simulink model "LCL_filter_blok_schem_S"  (R2021b)
settings: Solver=VariableStepAuto  StartTime=0.0  StopTime=Tsim  RelTol=1e-3
model workspace (MAT data in the model file):
  C = sym
  C.s = 'symobj::fromString("eJytU0tOwzAQddqUryqBBEJ0FQlOwAnKZ8MSumMTOWQogxxHZJyi7DgFd4JTYU8r6rhpxaKWXjKacd6bebH7QoieEJ9f9h33o4F9jUdivvo2PlnEdo/Yd6CGJBFONadb9SuHD8AqT2ayQpkpSLQsgJKaIE9QJ9QUZfZ2VxdFc5+DNviCUAlfsxdwxg6vpcpt/szbM+qIw375W1KlCfI7DmRyhRlrH4jlGjoQmElTXCuUBDSf89zT+BGttVZ/1yH9c6tVO3VYa8eSc9A5U53ZtsbfXhOHG/rgeVN4r6Vi7kvPu4tFHHV46fPHAeeeA5VqBuxiy0Ou3UjC5wmYgOco2MvzVOA6a/EzHtMVf32uYTCLXzsOdPhfoDYwZYdXtZ62p8XzV9Jgqbvneki3d+n+e5A2XSw/7w5CdGsfvwMla0g=", 2)'
  C.Digits = 32
  Cx = 3
  F = tf
  F.IOSize_ = [1 1]
  F.Data_ = ltipack.tfdata
  F.Data_.num = {[0 6e-06 0 0 0]}
  F.Data_.den = {[-3e-09 -9e-06 0.06 0.0002 1]}
  F.Data_.Delay.Input = 0
  F.Data_.Delay.Output = 0
  F.Data_.Delay.IO = 0
  F.Data_.Ts = 0
  I2 = sym
  I2.s = 'symobj::fromString("eJytVEtOwzAQdZqEfmgpf0RXkeAC9ATls0FiQys2bKKUmGLkJCVOWmXHKbgTXApiN1Bn4kRUraWRPePJm3nPdnSEUA2h9490NnTNTKdBDy2Gnq4Ps3Wag5rcWMIcxsjEF+Hcfp/bHJPQtWZOSJwxxZbveJhZMcOuRXyLJV4wfr2JPS+5dbEfkWeCQyTXrAFMg9tLQN00fiLl9BRr2K/4ltEgAvEtbixyKRmL2i20HB1uDEejxLukxGGYLXieSjW+UG6U1q9zs//Uyu0dcSuVY4lpKjnF47StwafUxHZFH4Kvjd9ihwrsc0m7s2ytKbSU8Q2A2eDGAjrDQsWchmLvymHkaYQjgLMLcgWfEPPOcvjChnZBXxmrA7jIe3ugjjgL4kd4IhQu1nrcXC3BP3QiEvhqXvf25h7dfy9S1cP6zamDHN6YaXsxjYp1+YXRrotxYXcXJfG+Guch36v6Ak+DefazKHyfPVIdLYeWOVrFoTalvYaS+5TGrNhb1cNYXNwS/sN+DstQYMn+FvC7wG9JWDAXYpkK7CpdZL8Ota1l8woYLYhhLDFycX6g3+lYg9sB8HeA3wb+8Zo6Qq2qzqy9wVqQV3fF85D9/TX6gpxVfcl+D+r/AxkWrVk=", 2)'
  I2.Digits = 32
  L1 = sym
  L1.s = 'symobj::fromString("eJytU8tOwzAQ3DYpT1UCCYToKRL8AHxBQVyQuJTeuEQOWYqRk4isU5QbX8E/wVdhbyvqOGnFoZZGWXmdmZ1JHABAH+DzyzzDoDcwj/EIFisw9cmyNmdg34JqEkRylvN2o39t8YGyTKO5KKVIFEa5yJCiijCNZB5RnRXJ212VZfV9irmWLxJLcDX7Hmdo8Vqo1OyfOWdGHbU/L79LqtDe/o4F6VTJhLUPYLWGFoR6Wmc3SgpCWvg8dzR+oLHW6u9axH9pNXqnFmvjWHEOOj1ViRlr/O0McbhhDvYb43slFHNfOtldLOteR5Yuf+hx7llQoebIKTYy5N6tIPk8Re3xHHln2U+JdrIGP+MxbuXrcg09L27v2NPhbyFzjTNOuK31tD0t9l8KLYu829ck3t6l+++PtOlitQZ8uAL4BQPqa4Q=", 2)'
  L1.Digits = 32
  L1x = 0.01
  L2 = sym
  L2.s = 'symobj::fromString("eJytU8tOwzAQdNuUpyqBBEL0FAm+gC8oiAsSF+iNS+SQpSxyHJF1inLjK/gn+CrsbUUdJ6041NIoK68zszOJB0KIvhCfX/YZDXpD+5iMxWINbH2yrO0Zse9ANUkinGnebvSvHD4AyyyeyxJlqiDWMgeKK4IsRh1TnRfp222V5/VdBtrgC0IpfM1+wBk5vBYqs/tn3plxRx3Oy++SKkywv+NAJlOYsvaBWK2RA4GZ1vm1QklAC5/nnsaPaKy1+rsOyV9ajd6pw9o4VpzDTk9VaseafHtDHG6Yg/0m8F5JxdyXXnYXy7rXkaXPHwWcew5UqDlwio0MuXcjCZ+nYAKeo+As+ynBTdbgZzwmrXx9rlHgxe8dBzr8LVAbmHHCba2n7Wmx/1IaLHS3r4dke5fuvz/SpovVGvDeXuVfA+1rhQ==", 2)'
  L2.Digits = 32
  L2x = 0.01
  R1 = sym
  R1.s = 'symobj::fromString("eJytU8tOwzAQ3LYpT1UCCYToKRL8AHxBQVw4Qm9cIocsxchxRNYpyo2v4J/gq7C3FXWctOJQS6OsvM7MziQeAEAf4PPLPqNBb2gfkzEs1sDWJ8vanoF9B6pJEMmZ5u1G/9rhA2WZxXNRSpEqjLXIkeKKMIuljqnOi/Ttrsrz+j5DbeSLxBJ8zX7AGTm8Fiqz+2femXFHHc7L75IqTLC/40AmUzJl7QNYrZEDoZnW+Y2SgpAWPs89jR9orLX6uw7JX1qN3qnD2jhWnMNOT1Vqx5p8e0McbpiD/Sb4XgnF3JdedhfLuteRpc8fBZx7DlSoOXKKjQy5dytIPk/RBDxHwVn2U6KbrMHPeExa+fpco8CL3zsOdPhbSG1wxgm3tZ62p8X+S2Fkobt9PSTbu3T//ZE2Xax28FcAvwQCa4o=", 2)'
  R1.Digits = 32
  R1x = 50
  R2 = sym
  R2.s = 'symobj::fromString("eJytU8tOwzAQdNuUpyqBBEL0FAm+gC8oiAtH6K2XyCFLWeQ4IusU5cZX8E/wVdjbijpOWnGopVFWXmdmZxIPhBB9IT6/7DMa9Ib2MRmL5RrY+mxV2zPi0IFqkkQ417zd6N84fACWWbyQJcpUQaxlDhRXBFmMOqY6L9K3+yrP64cMtMEXhFL4mv2AM3J4LVRm9y+8M+OOOpyX3yVVmGB/z4FMpjBl7SOxXiMHAjOt81uFkoCWPi89jR/RWBv19x2Sv7QavXOHjXGsOYednqrUjjX59oY43jIH+03gvZKKua+97K5Wda8jS58/CjgPHKhQC+AUGxly704SPk/BBDwnwVn2U4KbrMHPeEpa+fpco8CL3zsNdPhboDYw54TbWrPdabH/UhosdLevx2R3l+6/P9K2i9UO3l7lXwQFa4s=", 2)'
  R2.Digits = 32
  R2x = 20
  Tchirp = 0.04
  Tsim = 0.05
  Tstep = 0.02
  U = sym
  U.s = 'symobj::fromString("eJytU0tOwzAQddqUryqBBEJ0FQlOwAkKYsMSKjZsIocMZZDjiIxTlB2n4E5wKuxpRR03rVjU0ktGM857My92XwjRE+Lzy77jfjSwr/FIzFffxieL2O4R+w7UkCTCqeZ0q37l8AFY5clMVigzBYmWBVBSE+QJ6oSaoszebuuiaO5y0AZfECrha/YCztjhtVS5zZ95e0Ydcdgvf0uqNEF+x4FMrjBj7QOxXEMHAjNpimuFkoDmc557Gj+itdbq7zqkf261aqcOa+1Ycg46Z6oz29b422vicEMfPG8K77VUzH3peXexiKMOL33+OODcc6BSzYBdbHnItRtJ+DwBE/AcBXt5ngpcZy1+xkO64q/PNQxm8WvHgQ7/C9QGpuzwqtbT9rR4/koaLHX3XPfp9i7dfw/Spovl591BiB7t4xcDbWta", 2)'
  U.Digits = 32
  UR2 = sym
  UR2.s = 'symobj::fromString("eJytVEtOwzAQddq0Da0q/iC6igQXoCconw0SG1qxYROlxBQjJymx0yo7TsGd4FIQu4E6EydQtZZG8YzHb+Y926kjhGoIvb2nX7NuNNLPoIcWo57OD7J5moO2hLGEuYyRSSDDufW+sDkmkWfP3Ii4Y4rtwPUxs2OGPZsENkv8cPxyHft+cuPhgJMngiOk1qwBTFPYc0i9NH6s5PQ0c9iv3MtoyEG8KYxxj5KxrN1Gy9EVxjAfJf4FJS7DbMHzRKnxiXKjtH5LmPOrVm7tUFipHEvMhpZTPE7bGnwoTXQq+pB8Hfwau1RinynanWZzQ6Olim8CTEsYC+kMSxVzGsq1S5eRxxHmAGcH5Eo+ERad5fClDZ2CvipWF3BR13ZBHXkWJOB4IhUu1nrYXC3JP3I5CQM9rztnc4/uvxep6mH95FggRzTWcPyY8mJdcWGMq2Jc2u15Sbyvjw+LcYl/n+egv9jTcJ79RAr7s8dbR8thZI5RcdjtPzWZ0pgVe6t6MAueC13UPEvBMDUYqt/U7C37CcBciNXQYFfpofotqGkt+66A0YEY5hIjFxcH+ZWONbjtA39b87hV/2hNHaFWVWfW3WAtyMta8TxUf2+NviBnXV+q34P6fwPdPq5b", 2)'
  UR2.Digits = 32
  Ux = 10
  Z = sym
  Z.s = 'symobj::fromString("eJzNWN1O1EAUntJdERXERIMgxlW440a5xJgsgiQkEiPcGBSbWTq7jOkfnRYoV1z6BL6TPpMJdqaFnZ6ZTncNFzSZtGdm+p2/75zOro0QmkDo4ld+b9lWO791F1Bx2fnz4/I534Om+GAZw4zRQSCmK+urfJwSGrudExxT3PNIJ8A+YZ2UEbdDgw7L/LD3YzP1/WzbJUFC+5TESNY5ATBbfByFnpvPz0l7FjTP0F7xLvPCBMzf4YMlrkd7Qvc9NLym+WAk2cv8dY9iRljh57yk4w+qXLX6J/lwrqNVWXvCR204hphtrU9pLzer+1sy4r7BDuGvQ45T7AnsZSl2S+WzpYmljN8CmHf5YKF3QkQUKzEUa+8xo4d7JAE4s2Cv8Ccm3LIKvhi7jhJfGWsa+CKvPQJ6RC5okJCBiLCqa//mdAn/Y5zQMND79dm5uaIblUimwrpyrGUgxP8Ums3HZugjECBByB2cxPRM2GgioYmQstwGOh7y8eEsikkeuDDYooS7irrPhnhC94shHtffyte7M0OYCqZIHnXFPCw+iLOTz9lIuZT3ZPmBodHYOkJvhDmjg4Tjvizn8wJDPwsbkGvImSCpQ/IAMXKsy9unVOAqeXZxgg3NBzYKgeXQPjLsKWzx8HnmhPEYjUyOr2WVd938ZX4ZuDTXVCdBGPGGu3iFWYPztKmOCx9xICjUlBuPlJ4qOmT5ucGvjmavqfnL/OI8mi0+kmtr20GfBjTJxvhAmD6ywj8J0xRDkz6YD+iDsGEDR5GXCRtG7SUrWhzqFqVWzxUxwkjRpdSDj/mm6wONBTBlW14DeVFja12PHsdH0U/yfG2lwSFq0AkPGyYe1PXM2YZeeBtk5aDi0n5f7rWXlxdyr5X95nNWHyl+mw5qso66+EI+rBjqR9vLcDxgjT02xsGACNsrvXSivBv4ug7kmTG5I8tvgfzuFnBibM4kWUTAPv6dbziHWH8bsEWeKDsncSjeH+U80pQXWeb7684iFti7rXm3LsdTmhwr/JP8quPZpLQG7ZmCvLX1+/alHsztfDV8vq7hK5xSrj3D8EN82/FTT3wiND3w4xtlXvSI8gembNe8oT4LPZGXsho9u4Weuvh/BfI3IB/oesaS88UB8bFBfKSYVWIEdatxWVX8PzDEA2I6QMZj+A7r8qDhXXPPjMLT8s8MJccbSPER5lheOxohHrL8HciHDVwu5zTcUXPRh9j/AGWyXjA=", 2)'
  Z.Digits = 32
  ZI3 = sym
  ZI3.s = 'symobj::fromString("eJzNWN1O1EAUntJFRAUx0SCIcRXvuFEuMSaLIAmJxAgxMSg2s9vZZUz/6LRAueLSJ/Cd9JlMsDMt7PTMdLpruGCSk86ZmX7n/3R2bYTQBELnv/Jny7Ym80dnERXDzucPy3l+Bk1zYhnDjNFBIJYr+6ucTgiN3fYxjinueqQdYJ+wdsqI26ZBm2V+2P2xmfp+tu2SIKF9SmIky5wAmC1Oh6Hn5uvz0plFzRzqK95lXpiA9VucWOJ6tCtk30HDMcOJkWQv89c9ihlhhZ0Lkow/qDJq5U9xcq68Vdl7xKnWHUPMSa1NaTdXq/NbUuKuQQ9hr0OOUuwJ7JeS75bLuaXxpYzfApi3ObHQOybCixUfir13mNHeHkkAzhw4K+yJCdesgi9o11H8K2PNAFvkvQdAjogFDRIyEB5WZe1fnyxhf4wTGgZ6uz4511d0oyaSqbAuDWsZEuJ/Cs3mtBn6CDhIJOQOTmJ6KnQ0JaEpIWV+Esi4z+n9aRST3HFhsEUJNxV1ngzxhOxnQzwuv5Xvd2aHMBVMETzqinVYfBBnJ1+zkTKU92T+nqHR2LqE3gjzjA4Sjvu8XM8LDP0sdECuIWYiSR2SO4iRI13cPqYCV4mzixNsaD6wUQgsh/aR4Uyhi4fPMieMx2hksn8tq3zq1i/yYcil+aY6CcKIN9ylS8wanMdNdVzYiAORQk2x8UhpqSJD5p8a7Gprzpqav5xfPI/mio/k2tp20KcBTbIxPhCmj6ywT8I0+dAkD8YD2iB02MBR5GVCh1F7yYoWh7pFqdXniqAwUmQp9eBjfujqQmMBTFmXV4Bf0uha16PHsVH0kzxeW2nQQw0y4WXDlAd1PXOuoRfeBF65qLi035d77cXFudxrZbv5mtVHit2mi5oso86/MB9WDPWj7WU4HrDGHhvjYECE7pVeOlE+Dfm6DvjZMXNH5t8A/u0NyImxcybJIgLO8e98wz3E+tuALeJE2RmJQ/H+KPeRprjIPD9fdxexwNltzbt1MZ7WxFjJP8muujybkvagPtMwb239uX2pB3M9XwznVzV8iVPytXcYfomfdPzUE58ITQ/88FpZFz2i/IEp67VgqM9CTuSlrEbObiGnzv9fAf8N8Ae6nrHsfHGAf2zgH8lnFR9B2apfVhX7Dwz+gJgO4PEYtsO6PGh419wzo/Ck/DNDifEGUmyEMZb3Dkfwh8x/B3wPxMpC1VhZOh0/qzr2/gEclVyL", 2)'
  ZI3.Digits = 32
  a = [-3e-06 -0.009 60 0.2 1000]
  b = [0.006 0 0 0]
  cit = sym
  cit.s = 'symobj::fromString("eJytU0tOwzAQdZqEryqBBEJ0FQlOwAkCYsMSuusmcshQjJwEMk6r7DgFd4LzcABsJ1DbTSoWtfTk8YzzZubF4xNCRoS8f8g98L1QbvGEtMuX9klnyztkXwEbpIhsXmi3Fb9SWAKrsmhBK0ZTDlFBc8CoRsgiVkTY5GX6clvneXOXQSHYE4OKmDlHDmeg8FzyTPrPjDuTHtutV3+LvBSOf0cBRcZZqnMfkNUaKyCIaZNfc0YRsO3z3MjxRaw1mH9XIflTy4qdKgzKseIMe3uqU1lW/GkUcbihDt1vAm815Zr70tDuorO9Hi1N/sDh3FPAki9Aq2hpqGM3FNnjFITDc+Tc1f1UoCqz+DUekjV9Ta6x04sZO3by6H/BCgFzrfB6rtn2cun+KypYWfT3dZ9sb+j++5A2DdZQblVYmOQ1FzZX/wN7LZfdMJsx9bC8boh8QySvO8h4HJj+39i3155/AKW1cyg=", 2)'
  cit.Digits = 32
  color = 'r'
  men = sym
  men.s = 'symobj::fromString("eJy1VN1OgzAULgOm0yxqojHuikSfwGsv5uKNl7o7b0iROmsKTE7Zwp1P4Tvpk+wttC1MSmGbJrPJCeX8fN85Hy02QqiD0Nu7eDq25YrHcICKZYv9cbkXOagnDXLAAHQSK3ctfiltTmgaejOcUhww4sU4IuBlQEKPxh7kURK83GRRlN+GJOb0iZIU6ZwdA9OR9pywUPhPtZxBy97sV9UCS7jh70oDHjIaKO49VK2+NCB8nEfXjGIgUMx5pnF8otpayb8jzf9RqxY7kbZSjgrTbZ0pC0Rbww+tif01fah5ffKaYaawLzTtzsu91aKlju8YmLvSIGEzolSsaahiIwz0cUy4gXNo5Kp5UiI7q+Eru/cb+upYfWMWPXZk8KhvQWNOJkrhJtfD9rjU/CnmNInb57rzt3fpfnuQ1l2sZU7XyJGNuf6UZVDHMnss8qKM8WZ/8mBZZb2jiaT8VllcvK8U3914uKfJvPyR6HVyHlvn7FRcNf/V33vQY71NvHaF39BAfuCFSPgS67/4nTX8MnE4Oljy1+oWxZv1DVG6i7I=", 2)'
  men.Digits = 32
  s = sym
  s.s = 'symobj::fromString("eJytU0tOwzAQddqUryqBBEJ0FQlOwAkKYsMSuusmcshQBjmOyDhF2XEK7gSnwp5W1HHTikUtPXk047yZ92L3hRA9IT6/7B73o4HdxiOxWH0bny1je0YcOlBDkghnmtOt+o3DB2CVJ3NZocwUJFoWQElNkCeoE2qKMnu7r4uiechBG3xBqITfsxdwxg6vpcpt/sI7M+qIw3n5W1KlCfJ7DmRyhRn3PhKrNXQgMJOmuFUoCWih89Lr8SNaa2P/fYf0z61W7dxhox0rzkGnpjqzY42/vSGOt8zBelN4r6Vi7mvPu6tlHHV46fPHAeeBA5VqDuxiy0Ou3UnC5wmYgOckOMt6KnCTtfgZT+mavz7XMNDi106DPvwvUBuYscPrvaa768X6K2mw1N26HtPdPbr/XqRtD8vPu4sQuUv/CwPla3g=", 2)'
  s.Digits = 32
  sim = 'HPF'
  u = sym
  u.s = 'symobj::fromString("eJzNVk9P1EAUn9JFXBXERAMixlW8cTEeMSaLIAkHYpSYGC/NLJ1dx7TTpdNFyomjn8DvpJ/JZJ15Xdjp63TKGg5M8tLOn/7ev997HZ8QMkfI+S/1bPnevHp010gxfPX+cPKuzpC2FplLKiUfCFgu7b/W8oPxNOyc0JTTXsQ6gsZMdkaShR0uOjKPk9733VEc5/shExnvc5YSU+ccwmxp+ZZEoVpfMc6sWd6xvfCtjJIMrd/SIrMw4j3QfYdMx6IWybLDPN6OOJVMFn4+NnT8IaVRq39BS3AZrdLeIy214Zhizlt9GvWUWd3fhhF3HXaAvwE7HtEIsF8asduYvHuWWJr4LYR5W4tMohMGUSzFEPbeUcmPDlmGcJbRWfAnZdqyEj7Ip6ASXxNrEfli7j1AeiAXXGRsABGu6vp6fbrA/5RmPBF2vz4G11d0VyWSq7AuHGs5CPE/heZr2U1iggIEhDygWcpPwUYXCV2ENOfzSMd9Le9PhylTgUvEHmfaVdJ9MsUD3c+meFp/S+13l6YwJUxIHg9hHRcfxjlQaz6pjMp35vyeo9H4NkLvJIrRItO4zyfrqsDIz8IGEjpyBiQNmAqQZMe2vH0YAW4lzyHNqKP54EYBWAHvE8eZwpaInuVBks7QyMz4et7kaVsfq+Hg0kpTnYhkqBvu+gVmDc5qUx0XPlIBFGrKTcQmnlZ0mPOnDr86lrOu5m/yS/NoufhJbm3tiz4XPMtn+EG4frLgn4HpiqFLH84H9gFs2KHDYZSDDVftJZtWHB4WpVbPFZBkWNFVqYeY6kOXFxoPYZq2vELzdYutdT16Fh+hn6h87Y3EEWnQiS8bLh7U9czlhl54E+aVi0rI+32z147H52avNf3Wa16fVPx2XdRMHXXxxXzYdNSPtZfRdCAbe2xKxYCB7aVeOjd5Ovi6jeZLM3LHnL9B87c3gBMzcybLhwyd0//5hnuI97cBG/LE5RlLE/j+KveRpryYc32+7i7iobP7lm/rcty25LjCP8OvOp4tGHvYnjbmrW8/t4p68IupzUX9ksv8wH6lvj/DtFpjG8GX4B/i7DE2", 2)'
  u.Digits = 32
  wmax = 100000
  wmaxchirp = 1000
  wmin = 10
  wminchirp = 10
settings Model: Creator=Ivan  LastModifiedBy=Ivan

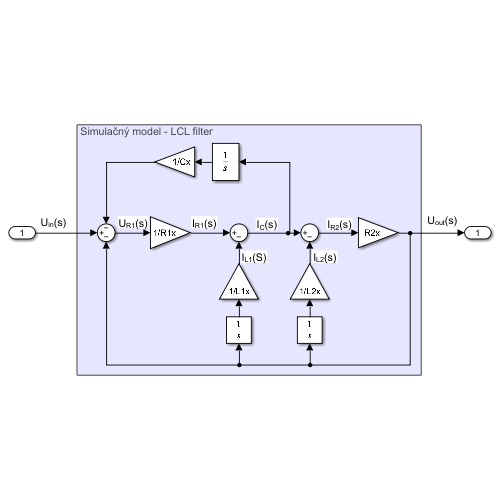
[thumbnail: Simulink's stored preview of the top-level diagram]
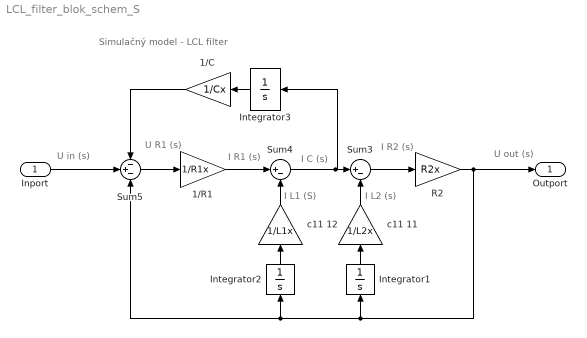
== system LCL_filter_blok_schem_S ==
  note: Simulačný model - LCL filter
  note: I R2 (s)
  note: I C (s)
  note: U out (s)
  note: U R1 (s)
  note: I L1 (S)
  note: I R1 (s)
  note: I L2 (s)
  note: U in (s)
  Inport : Inport
  1/C : Gain  Gain=1/Cx
  1/R1 : Gain  Gain=1/R1x
  Integrator1 : Integrator
  Integrator2 : Integrator
  Integrator3 : Integrator
  R2 : Gain  Gain=R2x
  Sum3 : Sum  Inputs=|+-  LockScale=on
  Sum4 : Sum  Inputs=|+-
  Sum5 : Sum  Inputs=-+-
  c11 11 : Gain  Gain=1/L2x
  c11 12 : Gain  Gain=1/L1x
  Outport : Outport
  wires:
  Integrator2/1 -> c11 12/1
  Integrator1/1 -> c11 11/1
  Sum5/1 -> 1/R1/1
  c11 12/1 -> Sum4/2
  1/C/1 -> Sum5/1
  R2/1 -> Outport/1, Sum5/3, Integrator2/1, Integrator1/1
  1/R1/1 -> Sum4/1
  Integrator3/1 -> 1/C/1
  Sum4/1 -> Integrator3/1, Sum3/1
  c11 11/1 -> Sum3/2
  Sum3/1 -> R2/1
  Inport/1 -> Sum5/2
